simulink subsystem "subsys_hauteur_aimants"  (R2021b)
settings: Solver=VariableStepAuto  StartTime=0.0  StopTime=10.0  RelTol=1e-3
settings Model: Creator=antho  LastModifiedBy=alexi

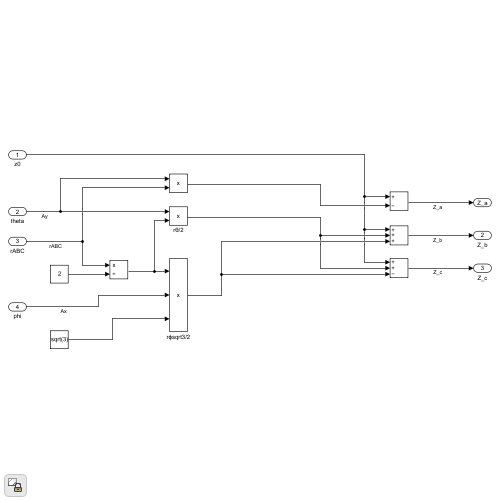
[thumbnail: Simulink's stored preview of the top-level diagram]
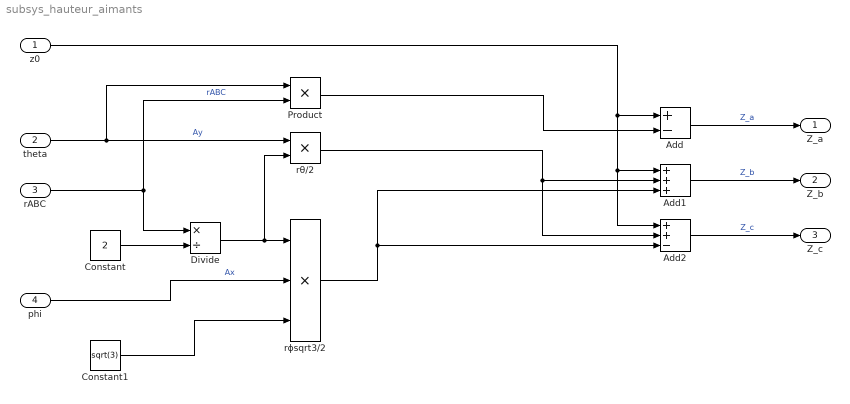
== system subsys_hauteur_aimants ==
  z0 : Inport
  theta : Inport  Port=2
  rABC : Inport  Port=3
  phi : Inport  Port=4
  Add : Sum  Inputs=+-
  Add1 : Sum  Inputs=+++
  Add2 : Sum  Inputs=++-
  Constant : Constant  Value=2
  Constant1 : Constant  Value=sqrt(3)
  Divide : Product  Inputs=*/
  Product : Product
  rθ/2 : Product
  rϕsqrt3/2 : Product  Inputs=3
  Z_a : Outport
  Z_b : Outport  Port=2
  Z_c : Outport  Port=3
  wires:
  Divide/1 -> rϕsqrt3/2/1, rθ/2/2
  Add2/1 -> Z_c/1  "Z_c"
  Add1/1 -> Z_b/1  "Z_b"
  Constant1/1 -> rϕsqrt3/2/3
  Add/1 -> Z_a/1  "Z_a"
  rABC/1 -> Divide/1, Product/2  "rABC"
  Product/1 -> Add/2
  rϕsqrt3/2/1 -> Add1/3, Add2/3
  Constant/1 -> Divide/2
  phi/1 -> rϕsqrt3/2/2  "Ax"
  z0/1 -> Add2/1, Add1/1, Add/1
  rθ/2/1 -> Add2/2, Add1/2
  theta/1 -> rθ/2/1, Product/1  "Ay"
